simulink model "z334b"  (Simulink 7.1)
settings: Solver=ode45  StartTime=-5.0  StopTime=10.0  RelTol=1e-3
settings Model: Creator=mestar  LastModifiedBy=mestar
settings DebuggingCC: SolverPrmCheckMsg=none

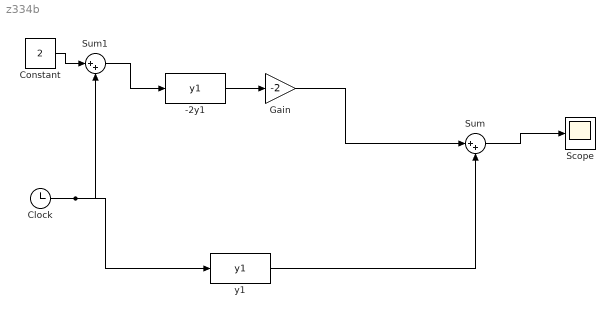
== system z334b ==
  -2y1 : MATLABFcn  MATLABFcn=y1
  Clock : Clock
      settings: Decimation=10
  Constant : Constant  Value=2  OutDataType=sfix(16)  OutScaling=2^0
  Gain : Gain  Gain=-2  ParameterDataType=sfix(16)  ParameterScaling=2^0  OutDataType=sfix(16)  OutScaling=2^0
  Scope : Scope
  Sum : Sum  Inputs=|++  OutDataType=sfix(16)  OutScaling=2^0
  Sum1 : Sum  Inputs=|++  OutDataType=sfix(16)  OutScaling=2^0
  y1 : MATLABFcn  MATLABFcn=y1
  wires:
  -2y1/1 -> Gain/1
  Clock/1 -> y1/1, Sum1/2
  Gain/1 -> Sum/1
  Sum/1 -> Scope/1
  y1/1 -> Sum/2
  Constant/1 -> Sum1/1
  Sum1/1 -> -2y1/1
